simulink model "cstr"  (Simulink 6.3)
settings: Solver=ode45  StartTime=0.0  StopTime=1000.0  RelTol=1e-3
settings Model: Creator=mbharadw  LastModifiedBy=mbharadw  ExtModeTrigMode=oneshot  ExtModeArmWhenConnect=off  StrictBusMsg=None
settings DataIOCC: LimitDataPoints=off
settings OptimizationCC: BlockReduction=off  BooleanDataType=off
settings DebuggingCC: SolverPrmCheckMsg=none
settings HardwareCC: TargetUnknown=on

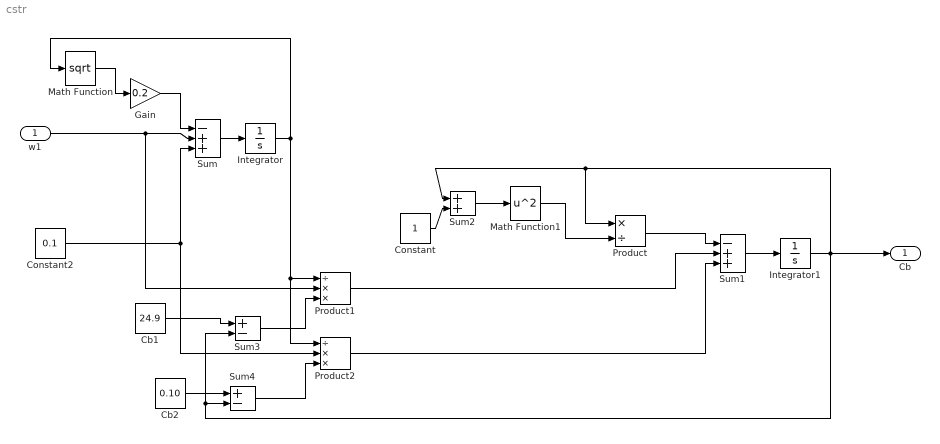
== system cstr ==
  w1 : Inport
  Cb1 : Constant  Value=24.9
  Cb2 : Constant  Value=0.10
  Constant : Constant
  Constant2 : Constant  Value=0.1
  Gain : Gain  Gain=0.2  SaturateOnIntegerOverflow=on
  Integrator : Integrator  InitialCondition=30  LimitOutput=on  LowerSaturationLimit=1
  Integrator1 : Integrator  InitialCondition=22
  Math Function : Math  Operator=sqrt  SaturateOnIntegerOverflow=on
  Math Function1 : Math  Operator=square  SaturateOnIntegerOverflow=on
  Product : Product  Inputs=*/  SaturateOnIntegerOverflow=on  RndMeth=Zero  InputSameDT=on
  Product1 : Product  Inputs=/**  SaturateOnIntegerOverflow=on  RndMeth=Zero  InputSameDT=on
  Product2 : Product  Inputs=/**  SaturateOnIntegerOverflow=on  RndMeth=Zero  InputSameDT=on
  Sum : Sum  Inputs=-++  SaturateOnIntegerOverflow=on  InputSameDT=on
  Sum1 : Sum  Inputs=-++  SaturateOnIntegerOverflow=on  InputSameDT=on
  Sum2 : Sum  SaturateOnIntegerOverflow=on  InputSameDT=on
  Sum3 : Sum  Inputs=+-  SaturateOnIntegerOverflow=on  InputSameDT=on
  Sum4 : Sum  Inputs=+-  SaturateOnIntegerOverflow=on  InputSameDT=on
  Cb : Outport
  wires:
  Sum/1 -> Integrator/1
  Gain/1 -> Sum/1
  Math Function/1 -> Gain/1
  Integrator/1 -> Math Function/1, Product1/1, Product2/1
  Cb1/1 -> Sum3/1
  Cb2/1 -> Sum4/1
  Sum3/1 -> Product1/3
  Sum4/1 -> Product2/3
  Constant/1 -> Sum2/2
  Sum2/1 -> Math Function1/1
  Sum1/1 -> Integrator1/1
  Math Function1/1 -> Product/2
  Product/1 -> Sum1/1
  Product1/1 -> Sum1/2
  Product2/1 -> Sum1/3
  w1/1 -> Sum/2, Product1/2
  Constant2/1 -> Sum/3, Product2/2
  Integrator1/1 -> Sum3/2, Sum4/2, Sum2/1, Product/1, Cb/1
